simulink model "Aufg_1KMod_TRY"  (R2020a)
settings: Solver=VariableStepAuto  StartTime=t_start  StopTime=t_end  FixedStep=dt_sim  RelTol=1e-3  EnableMultiTasking=on
libraries: carnot x3
settings Model: Creator=schabbach  LastModifiedBy=schabbach
settings SolverCC: AutoInsertRateTranBlk=on
settings DataIOCC: SaveFormat=Array  SaveOutput=off  SignalLogging=off  DSMLogging=off  SaveTime=off  ReturnWorkspaceOutputs=off  TimeSaveName=tsim
settings OptimizationCC: LifeSpan=inf
settings DebuggingCC: UnderspecifiedInitializationDetection=Classic  MergeDetectMultiDrivingBlocksExec=none  SolverPrmCheckMsg=warning  StateNameClashWarn=warning  SFUnexpectedBacktrackingDiag=warning  SFNoUnconditionalDefaultTransitionDiag=warning  SFExecutionAtInitializationDiag=none  ArithmeticOperatorsInVariantConditions=warning
settings HardwareCC: ProdBitPerPointer=32  ProdBitPerSizeT=32  ProdBitPerPtrDiffT=32  ProdLargestAtomicFloat=None  ProdIntDivRoundTo=Undefined  ProdEndianess=Unspecified  ProdWordSize=32  ProdHWDeviceType=32-bit Generic
settings ModelReferenceCC: PropagateSignalLabelsOutOfModel=off
settings SFSimCC: SimUseLocalCustomCode=off  CustomCodeUndefinedFunction=UseInterfaceOnly
settings RTWCC: RTWUseLocalCustomCode=off
settings CodeAppCC: StateflowObjectComments=on
settings GRTTargetCC: TargetLangStandard=C89/C90 (ANSI)
settings ConfigComp: CovMetricSettings=dw  CovHtmlReporting=on  CovSaveCumulativeToWorkspaceVar=on  CovSaveSingleToWorkspaceVar=on  CovExternalEMLEnable=off

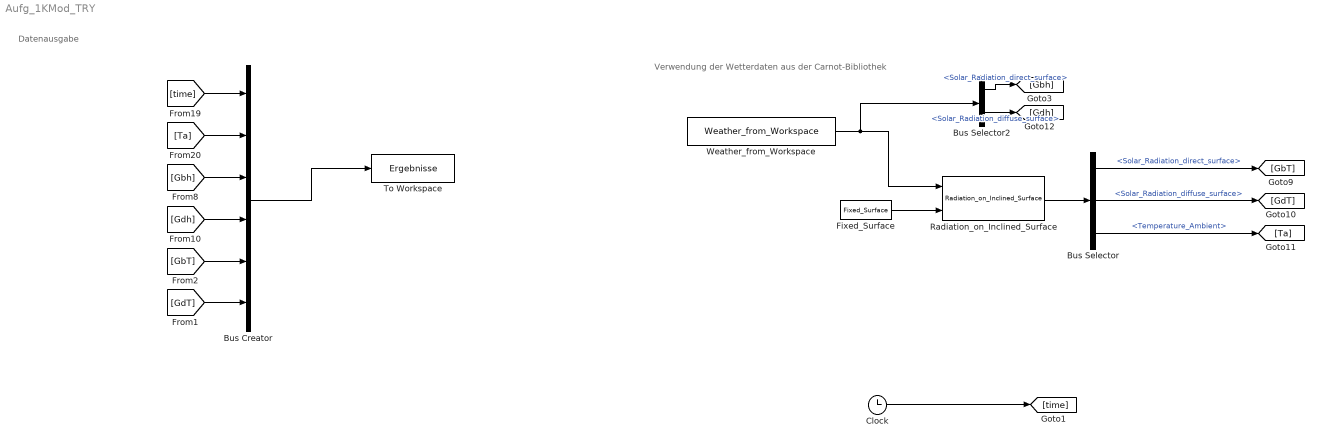
== system Aufg_1KMod_TRY ==
  note: Datenausgabe
  note: Verwendung der Wetterdaten aus der Carnot-Bibliothek
  Bus Creator : BusCreator  Inputs=6
  Bus Selector : BusSelector  OutputSignals=Solar_Radiation_direct_surface,Solar_Radiation_diffuse_surface,Temperature_Ambient
  Bus Selector2 : BusSelector  OutputSignals=Solar_Radiation_direct_surface,Solar_Radiation_diffuse_surface
  Clock : Clock
  Fixed_Surface : carnot/Weather/Fixed_Surface  colangle=slope  colazi=azimuth  colrot=0
      settings: SourceProductName=Carnot
  Radiation_on_Inclined_Surface : carnot/Weather/Radiation_on_Inclined_Surface  sky=Perez 1990  reflect=0.2
      settings: SourceProductName=Carnot
  To Workspace : ToWorkspace  VariableName=Ergebnisse  SampleTime=sampletime
      settings: Save2DSignal=2-D array (concatenate along first dimension)
  Weather_from_Workspace : carnot/Weather/Weather_from_Workspace  file=DE_TRY2010_07_averageYear
      settings: SourceProductName=Carnot
  wires:
  Bus Creator/1 -> To Workspace/1
  Fixed_Surface/1 -> Radiation_on_Inclined_Surface/2
  Weather_from_Workspace/1 -> Bus Selector2/1, Radiation_on_Inclined_Surface/1
  Radiation_on_Inclined_Surface/1 -> Bus Selector/1
  Bus Selector/1 -> [GbT]  "<Solar_Radiation_direct_surface>"
  Bus Selector/2 -> [GdT]  "<Solar_Radiation_diffuse_surface>"
  Bus Selector/3 -> [Ta]  "<Temperature_Ambient>"
  Bus Selector2/1 -> [Gbh]  "<Solar_Radiation_direct_surface>"
  Bus Selector2/2 -> [Gdh]  "<Solar_Radiation_diffuse_surface>"
  [time] -> Bus Creator/1
  [Ta] -> Bus Creator/2
  [Gbh] -> Bus Creator/3
  [Gdh] -> Bus Creator/4
  [GbT] -> Bus Creator/5
  [GdT] -> Bus Creator/6
  Clock/1 -> [time]
